simulink model "test_case_generator_BSC"  (R2024b)
settings: Solver=ode4  StartTime=0.0  StopTime=10.0  FixedStep=0.01  RelTol=1e-3  EnableMultiTasking=on
libraries: SignalEditorBlockLib x1
settings Model: Creator=nctzv8  LastModifiedBy=voillat
settings SolverCC: AlgebraicLoopSolver=TrustRegion
settings DataIOCC: LimitDataPoints=on
settings OptimizationCC: LifeSpan=inf
settings DebuggingCC: UnconnectedInputMsg=warning  UnconnectedOutputMsg=warning  UnconnectedLineMsg=warning  AllowSymbolicDim=off  SFUnexpectedBacktrackingDiag=warning  SFNoUnconditionalDefaultTransitionDiag=warning  SFExecutionAtInitializationDiag=none  ArithmeticOperatorsInVariantConditions=warning
settings ModelReferenceCC: EnableRefExpFcnMdlSchedulingChecks=on  PropagateSignalLabelsOutOfModel=off
settings SFSimCC: SimUseLocalCustomCode=off  CustomCodeUndefinedFunction=UseInterfaceOnly
settings RTWCC: RTWUseLocalCustomCode=off  GPUComputeCapability=3.5
settings CodeAppCC: StateflowObjectComments=on
settings GRTTargetCC: TargetLangStandard=C89/C90 (ANSI)
settings ConfigComp: CovMetricSettings=dw  CovSaveCumulativeToWorkspaceVar=on  CovSaveSingleToWorkspaceVar=on  CovExternalEMLEnable=off

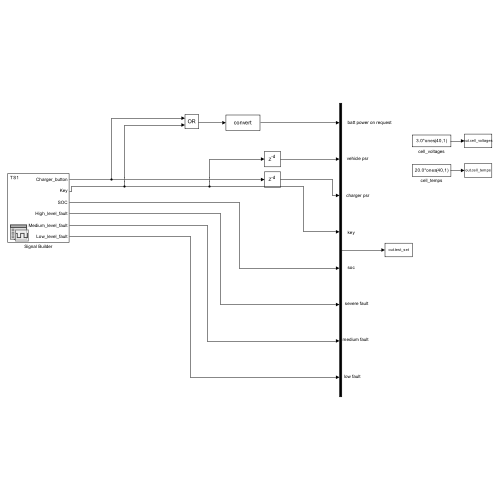
[thumbnail: Simulink's stored preview of the top-level diagram]
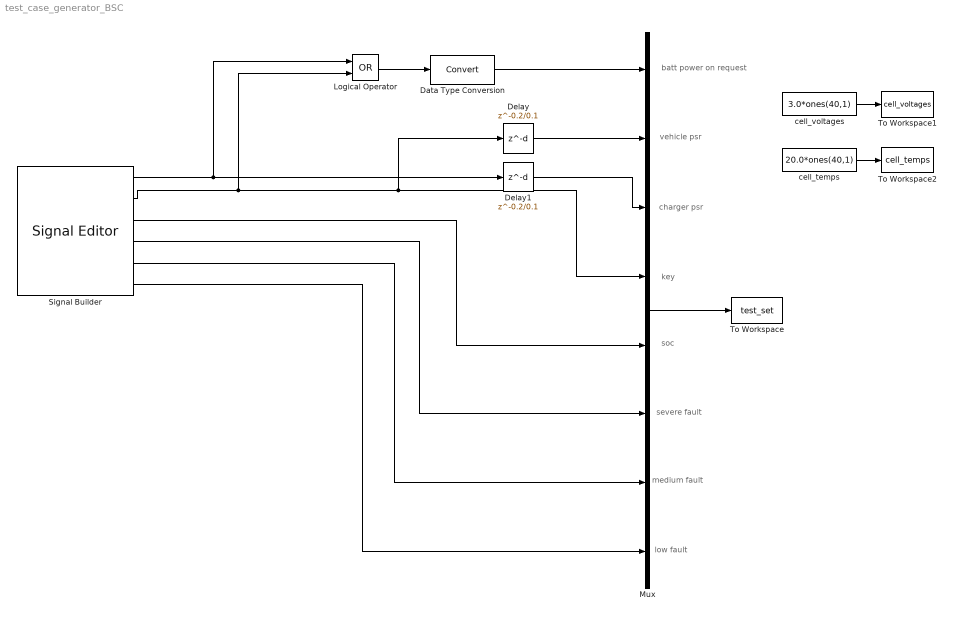
== system test_case_generator_BSC ==
  note: low fault
  note: medium fault
  note: severe fault
  note: soc
  note: charger psr
  note: key
  note: vehicle psr
  note: batt power on request
  Data Type Conversion : DataTypeConversion  SaturateOnIntegerOverflow=off  RndMeth=Floor
  Delay : Delay  DelayLength=0.2/0.1
  Delay1 : Delay  DelayLength=0.2/0.1
  Logical Operator : Logic  Operator=OR  AllPortsSameDT=off  OutDataTypeStr=boolean
  Mux : Mux  Inputs=8
  Signal Builder : SignalEditorBlockLib/Signal Editor  FileName=SignalBuilder.mat  ActiveScenario=TS1  ActiveSignal=Low_level_fault  IsBus=off  OutputBusObjectStr=Bus: BusObject  SampleTime=0  OutputAfterFinalValue=Extrapolation  Unit=inherit  PreserveSignalName=on  ApplySigPropsToAllScenarios=on  ApplySigPropsToAllSignals=off
  To Workspace : ToWorkspace  VariableName=test_set  SaveFormat=Timeseries  SampleTime=-1
  To Workspace1 : ToWorkspace  VariableName=cell_voltages  SaveFormat=Timeseries  SampleTime=-1
  To Workspace2 : ToWorkspace  VariableName=cell_temps  SaveFormat=Timeseries  SampleTime=-1
  cell_temps : Constant  Value=20.0*ones(40,1)
  cell_voltages : Constant  Value=3.0*ones(40,1)
  wires:
  Mux/1 -> To Workspace/1
  Signal Builder/3 -> Mux/5
  cell_voltages/1 -> To Workspace1/1
  cell_temps/1 -> To Workspace2/1
  Data Type Conversion/1 -> Mux/1
  Delay/1 -> Mux/2
  Signal Builder/4 -> Mux/6
  Signal Builder/5 -> Mux/7
  Signal Builder/6 -> Mux/8
  Signal Builder/1 -> Logical Operator/1, Delay1/1
  Signal Builder/2 -> Logical Operator/2, Delay/1, Mux/4
  Logical Operator/1 -> Data Type Conversion/1
  Delay1/1 -> Mux/3
